simulink model "GbxRe"  (R2020b)
settings: configuration reference "gen_config" (kept outside this file)
undefined symbols (not defined in the file): GbxRe_facGbxReRatio_C
settings Model: DataDictionary=Hybrid_vehicle.sldd  SimulationMode=accelerator  Creator=Georg  LastModifiedBy=jy
settings ConfigSetRef: SourceName=gen_config

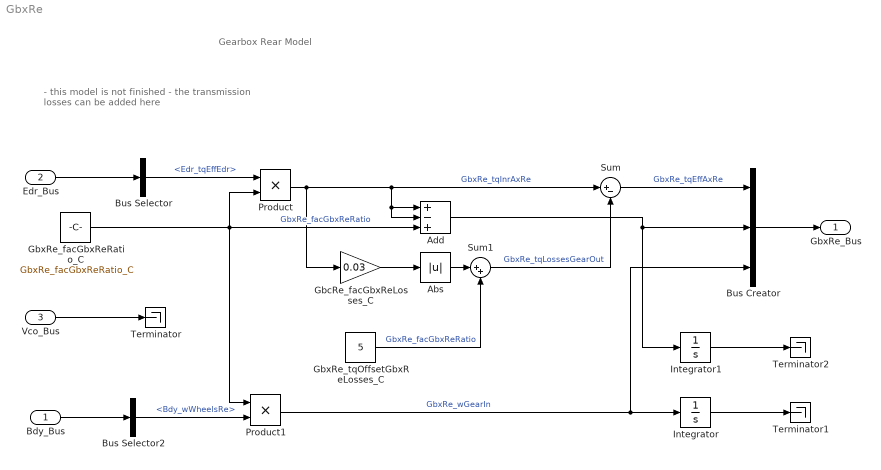
== system GbxRe ==
  note: Gearbox Rear Model
  note: - this model is not finished
      | - the transmission losses can be added here
  Bdy_Bus : Inport  OutDataTypeStr=Bus: BDY_BUS
  Edr_Bus : Inport  Port=2  OutDataTypeStr=Bus: EDR_BUS
  Vco_Bus : Inport  Port=3  OutDataTypeStr=Bus: VCO_BUS
  Abs : Abs
  Add : Sum  Inputs=+-+
  Bus Creator : BusCreator  Inputs=3  OutDataTypeStr=Bus: GBXRE_BUS
  Bus Selector : BusSelector  OutputSignals=Edr_tqEffEdr
  Bus Selector2 : BusSelector  OutputSignals=Bdy_wWheelsRe
  GbcRe_facGbxReLosses_C : Gain  Gain=0.03
  GbxRe_facGbxReRatio_C : Constant  Value=GbxRe_facGbxReRatio_C  SampleTime=-1
  GbxRe_tqOffsetGbxReLosses_C : Constant  Value=5
  Integrator : Integrator
  Integrator1 : Integrator
  Product : Product
  Product1 : Product
  Sum : Sum  Inputs=|+-
  Sum1 : Sum  Inputs=|++
  Terminator : Terminator
  Terminator1 : Terminator
  Terminator2 : Terminator
  GbxRe_Bus : Outport  OutDataTypeStr=Bus: GBXRE_BUS  VectorParamsAs1DForOutWhenUnconnected=off
  wires:
  Bus Selector/1 -> Product/1  "<Edr_tqEffEdr>"
  Vco_Bus/1 -> Terminator/1
  Edr_Bus/1 -> Bus Selector/1
  Product/1 -> Add/2, Add/1, Sum/1, GbcRe_facGbxReLosses_C/1  "GbxRe_tqInrAxRe"
  Bdy_Bus/1 -> Bus Selector2/1
  Bus Creator/1 -> GbxRe_Bus/1
  Sum1/1 -> Sum/2  "GbxRe_tqLossesGearOut"
  Sum/1 -> Bus Creator/1  "GbxRe_tqEffAxRe"
  GbxRe_tqOffsetGbxReLosses_C/1 -> Sum1/2  "GbxRe_facGbxReRatio"
  Product1/1 -> Integrator/1, Bus Creator/3  "GbxRe_wGearIn"
  Bus Selector2/1 -> Product1/2  "<Bdy_wWheelsRe>"
  Abs/1 -> Sum1/1
  GbcRe_facGbxReLosses_C/1 -> Abs/1
  Integrator/1 -> Terminator1/1
  Integrator1/1 -> Terminator2/1
  GbxRe_facGbxReRatio_C/1 -> Add/3, Product/2, Product1/1  "GbxRe_facGbxReRatio"
  Add/1 -> Integrator1/1, Bus Creator/2
